simulink model "UFFR_ob"  (Simulink 8.3)
settings: Solver=ode45  StartTime=0.0  StopTime=10  RelTol=1e-3
settings Model: Creator=Administrator  LastModifiedBy=JimmyChen
settings DataIOCC: SignalLoggingSaveFormat=Dataset
settings DebuggingCC: UnderspecifiedInitializationDetection=Simplified  StateNameClashWarn=none
settings GRTTargetCC: CombineOutputUpdateFcns=on  GRTInterface=off

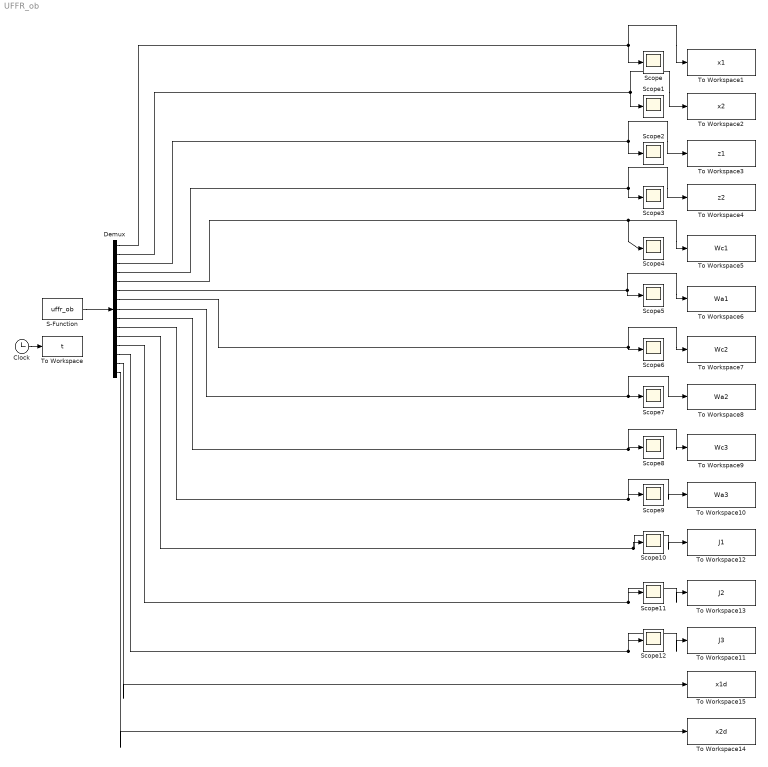
== system UFFR_ob ==
  Clock : Clock
  Demux : Demux  Outputs=15
  S-Function : S-Function  FunctionName=uffr_ob  EnableBusSupport=off
  Scope{,1..12} (13 alike) : Scope
      Scope10 settings: SaveName=ScopeData10
      Scope11 settings: SaveName=ScopeData11
      Scope12 settings: SaveName=ScopeData12
      Scope2 settings: SaveName=ScopeData2
      Scope3 settings: SaveName=ScopeData3
      Scope4 settings: SaveName=ScopeData4
      Scope5 settings: SaveName=ScopeData5
      Scope6 settings: SaveName=ScopeData6
      Scope7 settings: SaveName=ScopeData7
      Scope8 settings: SaveName=ScopeData8
      Scope9 settings: SaveName=ScopeData9
  To Workspace : ToWorkspace  VariableName=t  SaveFormat=Timeseries  SampleTime=-1
  To Workspace1 : ToWorkspace  VariableName=x1  SaveFormat=Timeseries  SampleTime=-1
  To Workspace10 : ToWorkspace  VariableName=Wa3  SaveFormat=Timeseries  SampleTime=-1
  To Workspace11 : ToWorkspace  VariableName=J3  SaveFormat=Timeseries  SampleTime=-1
  To Workspace12 : ToWorkspace  VariableName=J1  SaveFormat=Timeseries  SampleTime=-1
  To Workspace13 : ToWorkspace  VariableName=J2  SaveFormat=Timeseries  SampleTime=-1
  To Workspace14 : ToWorkspace  VariableName=x2d  SaveFormat=Timeseries  SampleTime=-1
  To Workspace15 : ToWorkspace  VariableName=x1d  SaveFormat=Timeseries  SampleTime=-1
  To Workspace2 : ToWorkspace  VariableName=x2  SaveFormat=Timeseries  SampleTime=-1
  To Workspace3 : ToWorkspace  VariableName=z1  SaveFormat=Timeseries  SampleTime=-1
  To Workspace4 : ToWorkspace  VariableName=z2  SaveFormat=Timeseries  SampleTime=-1
  To Workspace5 : ToWorkspace  VariableName=Wc1  SaveFormat=Timeseries  SampleTime=-1
  To Workspace6 : ToWorkspace  VariableName=Wa1  SaveFormat=Timeseries  SampleTime=-1
  To Workspace7 : ToWorkspace  VariableName=Wc2  SaveFormat=Timeseries  SampleTime=-1
  To Workspace8 : ToWorkspace  VariableName=Wa2  SaveFormat=Timeseries  SampleTime=-1
  To Workspace9 : ToWorkspace  VariableName=Wc3  SaveFormat=Timeseries  SampleTime=-1
  wires:
  S-Function/1 -> Demux/1
  Clock/1 -> To Workspace/1
  Demux/1 -> To Workspace1/1, Scope/1
  Demux/2 -> To Workspace2/1, Scope1/1
  Demux/3 -> To Workspace3/1, Scope2/1
  Demux/4 -> To Workspace4/1, Scope3/1
  Demux/5 -> Scope4/1, To Workspace5/1
  Demux/6 -> Scope5/1, To Workspace6/1
  Demux/7 -> To Workspace7/1, Scope6/1
  Demux/8 -> To Workspace8/1, Scope7/1
  Demux/9 -> To Workspace9/1, Scope8/1
  Demux/10 -> To Workspace10/1, Scope9/1
  Demux/11 -> To Workspace12/1, Scope10/1
  Demux/12 -> To Workspace13/1, Scope11/1
  Demux/13 -> To Workspace11/1, Scope12/1
  Demux/14 -> To Workspace15/1
  Demux/15 -> To Workspace14/1
